simulink model "TestDataLogging"  (R2019b)
settings: Solver=FixedStepAuto  StartTime=0.0  StopTime=100  RelTol=1e-3
InitFcn:
  | load('BusDefinitions.mat')
undefined symbols (not defined in the file or in its folder): codertarget, Ts
settings Model: ExtModeTrigDuration=80  Creator=Sankalp Bhan  LastModifiedBy=crbon
settings OptimizationCC: PassReuseOutputArgsThreshold=0  MaxStackSize=64
settings DebuggingCC: ParameterTunabilityLossMsg=error  ArithmeticOperatorsInVariantConditions=warning
settings HardwareCC: ProdBitPerPointer=32  ProdBitPerSizeT=32  ProdBitPerPtrDiffT=32  ProdLargestAtomicInteger=Long  ProdWordSize=32  ProdHWDeviceType=ARM Compatible->ARM 9  UseEmbeddedCoderFeatures=off
settings SFSimCC: SimUseLocalCustomCode=off  MATLABDynamicMemAlloc=off
settings RTWCC: SystemTargetFile=ert.tlc  HardwareBoard=PARROT Mambo  TLCOptions="-aInlineSetEventsForThisBaseRateFcn=TLC_FALSE -aSuppressMultiTaskScheduler=TLC_FALSE   -aRateBasedStepFcn=1"  TemplateMakefile=ert_default_tmf  GenerateReport=on  RTWUseLocalCustomCode=off  Toolchain=Sourcery G++ Lite GNU Toolchain for Drones  LaunchReport=on
settings CodeAppCC: ForceParamTrailComments=on  OperatorAnnotations=on  StateflowObjectComments=on
settings ERTTargetCC: ERTCustomFileBanners=off  MatFileLogging=on  SupportContinuousTime=on  SupportNonInlinedSFcns=on  RemoveResetFunc=off  ModelStepFunctionPrototypeControlCompliant=off

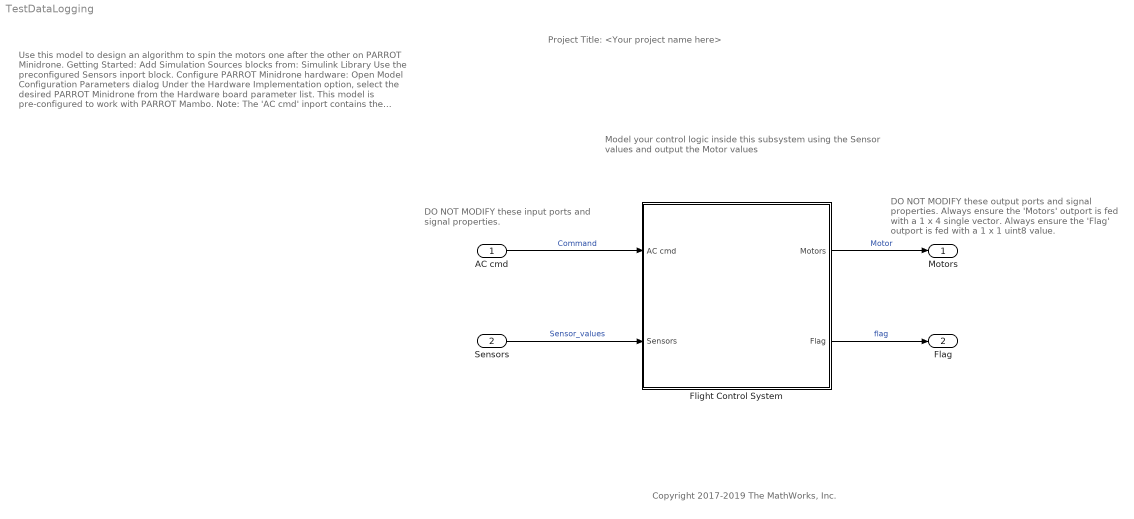
== system TestDataLogging ==
  note: Model your control logic inside this subsystem
      | using the Sensor values and output the
      | Motor values
  note: DO NOT MODIFY these output ports
      | and signal properties.
      |
      |
      |
      | Always ensure the 'Motors' outport
      | is fed with a 1 x 4 single vector.
      |
      |
      |
      |
      |
      | Always ensure the 'Flag' outport is
      | fed with a 1 x 1 uint8 value.
  note: DO NOT MODIFY these input
      | ports and signal properties.
  note: Copyright 2017-2019 The MathWorks, Inc.
  note: Use this model to design an algorithm to spin the motors one
      | after the other on PARROT Minidrone.
      |
      | Getting Started:
      |
      | Add Simulation Sources blocks from:
      | Simulink Library
      | Use the preconfigured Sensors inport block.
      |
      | Configure PARROT Minidrone hardware:
      |
      | Open Model Configuration Parameters dialog
      |
      | Under the Hardware Implementation option, select the desired
      | PARROT Minidrone from the Hardware board parameter list.
      |
      | This model is pre-configured to work with PARROT Mambo.
      |
      | Note:
      |
      | The 'AC cmd' inport contains the position and orientation
      | reference signals information.
      | The 'Sensors' inport contains data from accelerometer,
      | gyroscope, ultrasonic, pressure and optical flow data.
      | The 'Flag' outport can be used to model an error condition
      | which stops the drone.
      | The 'Motors' outport is fed with the speed values of the 4 motors.
      | Learn more:
      |
      | Simulink Subsystem
      | Simulink Buses
  note: Project Title: <Your project name here>
  AC cmd : Inport  OutDataTypeStr=Bus: CommandBus  BusOutputAsStruct=on
  Sensors : Inport  Port=2  OutDataTypeStr=Bus: SensorsBus  BusOutputAsStruct=on
  Flight Control System : Subsystem  InitFcn=codertarget.parrot.internal.fcsSubsystemCallback(gcb);
  Motors : Outport  OutDataTypeStr=single  PortDimensions=[1 4]  VectorParamsAs1DForOutWhenUnconnected=off
  Flag : Outport  Port=2  OutDataTypeStr=uint8  PortDimensions=1  VectorParamsAs1DForOutWhenUnconnected=off
  wires:
  Flight Control System/1(Motors) -> Motors/1  "Motor"
  AC cmd/1 -> Flight Control System/1(AC cmd)  "Command"
  Sensors/1 -> Flight Control System/2(Sensors)  "Sensor_values"
  Flight Control System/2(Flag) -> Flag/1  "flag"

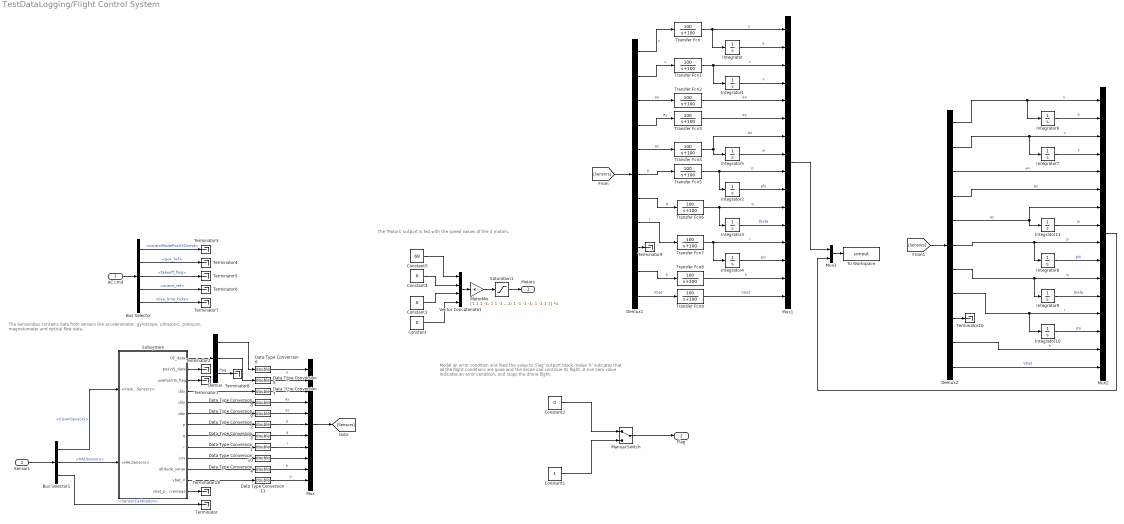
== system TestDataLogging/Flight Control System ==
  note: The 'Motors' outport is fed with the speed values of the 4 motors.
  note: Model an error condition and feed the value to 'Flag' outport block.
      | Value '0' indicates that all the flight conditions are good and the drone
      | can continue its flight.
      | A non-zero value indicates an error condition, and stops the drone
      | flight.
  note: The SensorsBus contains data from sensors like
      | accelerometer, gyroscope, ultrasonic, pressure,
      | magnetometer and optical flow data.
  AC cmd : Inport
  Sensors : Inport  Port=2
  Bus Selector : BusSelector  OutputSignals=controlModePosVSOrient,pos_ref,takeoff_flag,orient_ref,live_time_ticks
  Bus Selector1 : BusSelector  OutputSignals=VisionSensors,HALSensors,SensorCalibration
  Constant : Constant  Value=0  SampleTime=Ts
  Constant1 : Constant  OutDataTypeStr=uint8
  Constant2 : Constant  Value=0  OutDataTypeStr=uint8
  Constant3 : Constant  Value=0  SampleTime=Ts
  Constant4 : Constant  Value=0  SampleTime=Ts
  Constant5 : Constant  Value=68  SampleTime=Ts
  Data Type Conversion{1..11} (11 alike) : DataTypeConversion  OutDataTypeStr=double
  Demux : Demux  Outputs=3
  Demux1 : Demux  Outputs=11
  Demux2 : Demux  Outputs=11
  Integrator{,1..11} (12 alike) : Integrator
  Manual Switch : ManualSwitch
  MotorMix : Gain  Gain=[1 1 1 -1; 1 1 -1 1; 1 -1 -1 -1; 1 -1 1 1]  Multiplication=Matrix(K*u)
  Mux : Mux  Inputs=11
  Mux1 : Mux  Inputs=16
  Mux2 : Mux  Inputs=16
  Mux3 : Mux  Inputs=2
  Saturation1 : Saturate  UpperLimit=500  LowerLimit=0  OutDataTypeStr=single
  Subsystem : Subsystem
  Terminator{,1..10,18} (12 alike) : Terminator
  To Workspace : ToWorkspace  VariableName=simout  SaveFormat=Structure With Time  SampleTime=-1
  Transfer Fcn{,1..9} (10 alike) : TransferFcn  Numerator=[100]  Denominator=[1 100]
  Vector Concatenate1 : Concatenate  NumInputs=4
  Motors : Outport  VectorParamsAs1DForOutWhenUnconnected=off
  Flag : Outport  Port=2  VectorParamsAs1DForOutWhenUnconnected=off
  wires:
  AC cmd/1 -> Bus Selector/1
  Sensors/1 -> Bus Selector1/1
  Bus Selector/1 -> Terminator3/1  "<controlModePosVSOrient>"
  Bus Selector/2 -> Terminator4/1  "<pos_ref>"
  Bus Selector/3 -> Terminator5/1  "<takeoff_flag>"
  Bus Selector/4 -> Terminator6/1  "<orient_ref>"
  Bus Selector/5 -> Terminator7/1  "<live_time_ticks>"
  Manual Switch/1 -> Flag/1
  Constant2/1 -> Manual Switch/1
  Constant1/1 -> Manual Switch/2
  Vector Concatenate1/1 -> MotorMix/1
  Constant5/1 -> Vector Concatenate1/1
  Constant/1 -> Vector Concatenate1/4
  Constant4/1 -> Vector Concatenate1/2
  Constant3/1 -> Vector Concatenate1/3
  Saturation1/1 -> Motors/1
  Bus Selector1/1 -> Subsystem/1(<VisionSensors>)  "<VisionSensors>"
  Bus Selector1/2 -> Subsystem/2(<HALSensors>)  "<HALSensors>"
  Bus Selector1/3 -> Terminator/1  "<SensorCalibration>"
  Subsystem/1(OF_data) -> Demux/1
  Subsystem/4(ddx) -> Data Type Conversion7/1
  Subsystem/5(ddy) -> Data Type Conversion8/1
  Subsystem/6(ddz) -> Data Type Conversion9/1
  Subsystem/7(p) -> Data Type Conversion2/1
  Subsystem/9(r) -> Data Type Conversion1/1
  Subsystem/11(altitude_sonar) -> Data Type Conversion4/1
  Subsystem/12(vbat_V) -> Data Type Conversion11/1
  Subsystem/13(vbat_percentage) -> Terminator18/1
  Subsystem/8(q) -> Data Type Conversion3/1
  Mux/1 -> [Sensors]
  MotorMix/1 -> Saturation1/1
  Subsystem/3(usePosVIS_flag) -> Terminator1/1
  Subsystem/2(posVIS_data) -> Terminator2/1
  Demux/1 -> Data Type Conversion6/1
  Demux/2 -> Data Type Conversion5/1
  Demux/3 -> Terminator8/1  "flag"
  Subsystem/10(prs) -> Data Type Conversion10/1
  Data Type Conversion1/1 -> Mux/8  "r"
  Data Type Conversion2/1 -> Mux/6  "p"
  Data Type Conversion3/1 -> Mux/7  "q"
  Data Type Conversion4/1 -> Mux/10  "h"
  Data Type Conversion5/1 -> Mux/2  "v"
  Data Type Conversion6/1 -> Mux/1  "u"
  Data Type Conversion7/1 -> Mux/3  "ax"
  Data Type Conversion8/1 -> Mux/4  "ay"
  Data Type Conversion9/1 -> Mux/5  "az"
  Data Type Conversion10/1 -> Mux/9
  Data Type Conversion11/1 -> Mux/11  "V"
  [Sensors] -> Demux1/1
  Demux1/1 -> Transfer Fcn/1  "u"
  Demux1/2 -> Transfer Fcn1/1  "v"
  Demux1/4 -> Transfer Fcn3/1  "ay"
  Demux1/3 -> Transfer Fcn2/1  "ax"
  Demux1/7 -> Transfer Fcn6/1  "q"
  Demux1/8 -> Transfer Fcn7/1  "r"
  Demux1/6 -> Transfer Fcn5/1  "p"
  Demux1/5 -> Transfer Fcn4/1  "az"
  Demux1/9 -> Terminator9/1
  Demux1/10 -> Transfer Fcn8/1  "h"
  Demux1/11 -> Transfer Fcn9/1  "Vbat"
  Transfer Fcn/1 -> Integrator/1, Mux1/1  "u"
  Transfer Fcn2/1 -> Mux1/5  "ax"
  Transfer Fcn3/1 -> Mux1/6  "ay"
  Transfer Fcn6/1 -> Integrator3/1, Mux1/11  "q"
  Transfer Fcn5/1 -> Integrator2/1, Mux1/9  "p"
  Transfer Fcn7/1 -> Mux1/13, Integrator4/1  "r"
  Transfer Fcn4/1 -> Integrator5/1, Mux1/7  "az"
  Transfer Fcn8/1 -> Mux1/15  "h"
  Integrator4/1 -> Mux1/14  "psi"
  Integrator3/1 -> Mux1/12  "theta"
  Integrator2/1 -> Mux1/10  "phi"
  Integrator5/1 -> Mux1/8  "w"
  Integrator1/1 -> Mux1/4  "Y"
  Transfer Fcn1/1 -> Integrator1/1, Mux1/3  "v"
  Integrator/1 -> Mux1/2  "X"
  Mux1/1 -> Mux3/1
  Transfer Fcn9/1 -> Mux1/16  "Vbat"
  Demux2/5 -> Integrator11/1, Mux2/7  "az"
  Demux2/8 -> Mux2/13, Integrator10/1  "r"
  Mux2/1 -> Mux3/2
  Demux2/10 -> Mux2/15  "h"
  [Sensors] -> Demux2/1
  Demux2/7 -> Integrator9/1, Mux2/11  "q"
  Demux2/11 -> Mux2/16  "Vbat"
  Demux2/3 -> Mux2/5  "ax"
  Integrator8/1 -> Mux2/10  "phi"
  Integrator9/1 -> Mux2/12  "theta"
  Integrator10/1 -> Mux2/14  "psi"
  Demux2/4 -> Mux2/6  "ay"
  Demux2/9 -> Terminator10/1
  Demux2/6 -> Integrator8/1, Mux2/9  "p"
  Demux2/1 -> Integrator6/1, Mux2/1  "u"
  Integrator6/1 -> Mux2/2  "X"
  Integrator11/1 -> Mux2/8  "w"
  Integrator7/1 -> Mux2/4  "Y"
  Demux2/2 -> Integrator7/1, Mux2/3  "v"
  Mux3/1 -> To Workspace/1

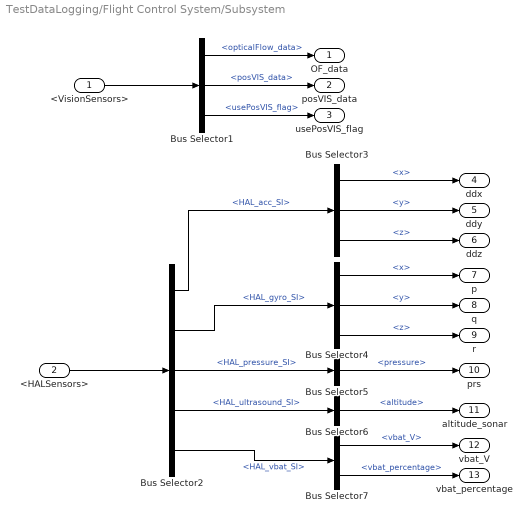
== system TestDataLogging/Flight Control System/Subsystem ==
  <VisionSensors> : Inport
  <HALSensors> : Inport  Port=2
  Bus Selector1 : BusSelector  OutputSignals=opticalFlow_data,posVIS_data,usePosVIS_flag
  Bus Selector2 : BusSelector  OutputSignals=HAL_acc_SI,HAL_gyro_SI,HAL_pressure_SI,HAL_ultrasound_SI,HAL_vbat_SI
  Bus Selector3 : BusSelector  OutputSignals=x,y,z
  Bus Selector4 : BusSelector  OutputSignals=x,y,z
  Bus Selector5 : BusSelector  OutputSignals=pressure
  Bus Selector6 : BusSelector  OutputSignals=altitude
  Bus Selector7 : BusSelector  OutputSignals=vbat_V,vbat_percentage
  OF_data : Outport  VectorParamsAs1DForOutWhenUnconnected=off
  posVIS_data : Outport  Port=2  VectorParamsAs1DForOutWhenUnconnected=off
  usePosVIS_flag : Outport  Port=3  VectorParamsAs1DForOutWhenUnconnected=off
  ddx : Outport  Port=4  VectorParamsAs1DForOutWhenUnconnected=off
  ddy : Outport  Port=5  VectorParamsAs1DForOutWhenUnconnected=off
  ddz : Outport  Port=6  VectorParamsAs1DForOutWhenUnconnected=off
  p : Outport  Port=7  VectorParamsAs1DForOutWhenUnconnected=off
  q : Outport  Port=8  VectorParamsAs1DForOutWhenUnconnected=off
  r : Outport  Port=9  VectorParamsAs1DForOutWhenUnconnected=off
  prs : Outport  Port=10  VectorParamsAs1DForOutWhenUnconnected=off
  altitude_sonar : Outport  Port=11  VectorParamsAs1DForOutWhenUnconnected=off
  vbat_V : Outport  Port=12  VectorParamsAs1DForOutWhenUnconnected=off
  vbat_percentage : Outport  Port=13  VectorParamsAs1DForOutWhenUnconnected=off
  wires:
  <VisionSensors>/1 -> Bus Selector1/1
  <HALSensors>/1 -> Bus Selector2/1
  Bus Selector1/1 -> OF_data/1  "<opticalFlow_data>"
  Bus Selector1/2 -> posVIS_data/1  "<posVIS_data>"
  Bus Selector1/3 -> usePosVIS_flag/1  "<usePosVIS_flag>"
  Bus Selector2/1 -> Bus Selector3/1  "<HAL_acc_SI>"
  Bus Selector2/2 -> Bus Selector4/1  "<HAL_gyro_SI>"
  Bus Selector2/3 -> Bus Selector5/1  "<HAL_pressure_SI>"
  Bus Selector2/4 -> Bus Selector6/1  "<HAL_ultrasound_SI>"
  Bus Selector2/5 -> Bus Selector7/1  "<HAL_vbat_SI>"
  Bus Selector3/1 -> ddx/1  "<x>"
  Bus Selector3/2 -> ddy/1  "<y>"
  Bus Selector3/3 -> ddz/1  "<z>"
  Bus Selector4/2 -> q/1  "<y>"
  Bus Selector4/1 -> p/1  "<x>"
  Bus Selector4/3 -> r/1  "<z>"
  Bus Selector5/1 -> prs/1  "<pressure>"
  Bus Selector6/1 -> altitude_sonar/1  "<altitude>"
  Bus Selector7/1 -> vbat_V/1  "<vbat_V>"
  Bus Selector7/2 -> vbat_percentage/1  "<vbat_percentage>"
